simulink model "simulink_svpwm"  (R2017b)
settings: Solver=FixedStepAuto  StartTime=0.0  StopTime=5  FixedStep=0.000064  RelTol=1e-3
model workspace (MAT data in the model file):
  TEST = [0 0 0 0 0 0 0 0 0 0 0 0 ... (737281 elements, 1x737281)]
libraries: powerlib x8, dspfdesign x3
settings Model: Creator=Administrator  LastModifiedBy=Administrator

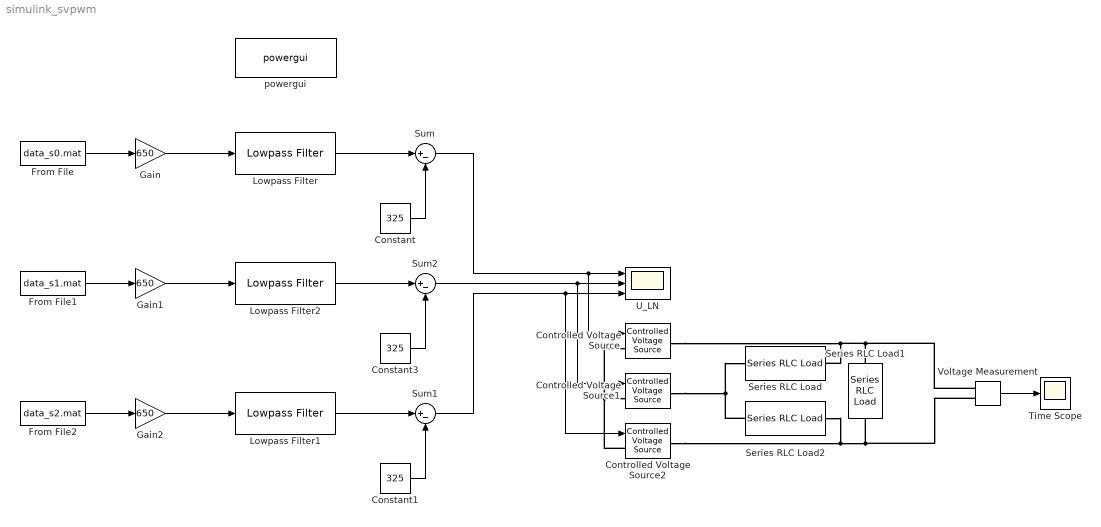
== system simulink_svpwm ==
  Constant : Constant  Value=325
  Constant1 : Constant  Value=325
  Constant3 : Constant  Value=325
  Controlled Voltage Source : powerlib/Electrical Sources/Controlled Voltage Source  Initialize=on  Source_Type=AC  Amplitude=0  Phase=0  Frequency=0  Measurements=None
  Controlled Voltage Source1 : powerlib/Electrical Sources/Controlled Voltage Source  Initialize=on  Source_Type=AC  Amplitude=0  Phase=0  Frequency=0  Measurements=None
  Controlled Voltage Source2 : powerlib/Electrical Sources/Controlled Voltage Source  Initialize=on  Source_Type=AC  Amplitude=0  Phase=0  Frequency=0  Measurements=None
  From File : FromFile  FileName=data_s0.mat
  From File1 : FromFile  FileName=data_s1.mat
  From File2 : FromFile  FileName=data_s2.mat
  Gain : Gain  Gain=650
  Gain1 : Gain  Gain=650
  Gain2 : Gain  Gain=650
  Lowpass Filter : dspfdesign/Lowpass Filter  FilterType=IIR  DesignForMinimumOrder=on  FilterOrder=50  PassbandFrequency=60  StopbandFrequency=1000  PassbandRipple=0.1  StopbandAttenuation=80  InheritSampleRate=off  SampleRate=44100  SimulateUsing=Interpreted execution  roundingMode=Floor  coeffsDataTypeStr=fixdt(1,16)
  Lowpass Filter1 : dspfdesign/Lowpass Filter  FilterType=IIR  DesignForMinimumOrder=on  FilterOrder=50  PassbandFrequency=60  StopbandFrequency=1000  PassbandRipple=0.1  StopbandAttenuation=80  InheritSampleRate=off  SampleRate=44100  SimulateUsing=Interpreted execution  roundingMode=Floor  coeffsDataTypeStr=fixdt(1,16)
  Lowpass Filter2 : dspfdesign/Lowpass Filter  FilterType=IIR  DesignForMinimumOrder=on  FilterOrder=50  PassbandFrequency=60  StopbandFrequency=1000  PassbandRipple=0.1  StopbandAttenuation=80  InheritSampleRate=off  SampleRate=44100  SimulateUsing=Interpreted execution  roundingMode=Floor  coeffsDataTypeStr=fixdt(1,16)
  Series RLC Load : powerlib/Elements/Series RLC Load  LConnTagsString=a  RConnTagsString=__new0  NominalVoltage=325  NominalFrequency=50  ActivePower=1  InductivePower=0  CapacitivePower=0  Setx0=off  InitialVoltage=0  SetiL0=off  InitialCurrent=0  Measurements=None  LoadType=constant Z
  Series RLC Load1 : powerlib/Elements/Series RLC Load  LConnTagsString=a  RConnTagsString=__new0  NominalVoltage=325  NominalFrequency=50  ActivePower=1  InductivePower=0  CapacitivePower=0  Setx0=off  InitialVoltage=0  SetiL0=off  InitialCurrent=0  Measurements=None  LoadType=constant Z
  Series RLC Load2 : powerlib/Elements/Series RLC Load  LConnTagsString=a  RConnTagsString=__new0  NominalVoltage=325  NominalFrequency=50  ActivePower=1  InductivePower=0  CapacitivePower=0  Setx0=off  InitialVoltage=0  SetiL0=off  InitialCurrent=0  Measurements=None  LoadType=constant Z
  Sum : Sum  Inputs=|+-
  Sum1 : Sum  Inputs=|+-
  Sum2 : Sum  Inputs=|+-
  Time Scope : Scope
  U_LN : Scope  NumInputPorts=3
  Voltage Measurement : powerlib/Measurements/Voltage Measurement  PhasorSimulation=off  OutputType=Complex  PSBequivalent=0
  powergui : powerlib/powergui  Priority=1  SimulationMode=Discrete  SampleTime=0.000064  frequency=60  Iterations=50  frequencyindice=0  Pbase=100e6  ErrMax=1e-4  UnitsV=kV  UnitsW=MW  buscounter=0  FunctionMessages=off  echomessages=off  EnableUseOfTLC=off  CurrentSourceSwitches=off  DisableSnubberDevices=off  DisableRonSwitches=off  DisableVfSwitches=off  DisplayEquations=off  SolverType=Tustin/Backward Euler (TBE)  Interpol=off  ExternalGateDelay=off  methode=off  Ts=100  x0status=blocks  SPID=off  SwTol=0  HookPort=off  RestoreLinks=warning  ResistiveCurrentMeasurement=off  Frange=[0:2:500]  Ylog=off  Xlog=on  ShowGrid=off  save=off  variable=ZData  structure=0  ZoomFFT=off  StartTime=0.0  cycles=1  DisplayStyle=1  fundamental=60  FreqAxis=off  MaxFrequency=1000  frequencyindicesteady=1  RmsSteady=1  display=off
  wires:
  From File/1 -> Gain/1
  Lowpass Filter/1 -> Sum/1
  Constant/1 -> Sum/2
  Gain/1 -> Lowpass Filter/1
  Gain1/1 -> Lowpass Filter2/1
  Constant3/1 -> Sum2/2
  From File1/1 -> Gain1/1
  Sum2/1 -> U_LN/2, Controlled Voltage Source1/1
  Lowpass Filter2/1 -> Sum2/1
  Gain2/1 -> Lowpass Filter1/1
  Constant1/1 -> Sum1/2
  From File2/1 -> Gain2/1
  Sum1/1 -> U_LN/3, Controlled Voltage Source2/1
  Lowpass Filter1/1 -> Sum1/1
  Sum/1 -> Controlled Voltage Source/1, U_LN/1
  Voltage Measurement/1 -> Time Scope/1
  connections:
  Controlled Voltage Source2/LConn1 -- Controlled Voltage Source/LConn1 -- Controlled Voltage Source1/LConn1
  Series RLC Load2/RConn1 -- Voltage Measurement/LConn2 -- Series RLC Load1/RConn1 -- Controlled Voltage Source2/RConn1
  Series RLC Load1/LConn1 -- Voltage Measurement/LConn1 -- Controlled Voltage Source/RConn1 -- Series RLC Load/RConn1
  Controlled Voltage Source1/RConn1 -- Series RLC Load/LConn1 -- Series RLC Load2/LConn1
